simulink model "Pendulo_doble"  (R2023a)
settings: Solver=ode23  StartTime=0.0  StopTime=15  RelTol=1e-3
values from neighbouring files (symbols this model uses):
  g = 9.81    [Condiciones.mat]
  L1 = 0.3    [Condiciones.mat]
  L2 = 0.25    [Condiciones.mat]
  m1 = 0.2    [Condiciones.mat]
  m2 = 0.1    [Condiciones.mat]
settings Model: Creator=andre  LastModifiedBy=andre

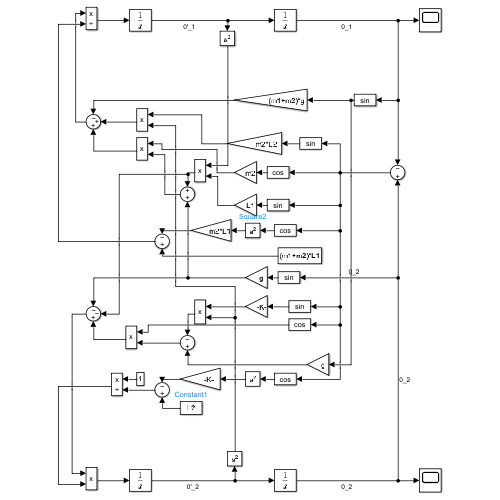
[thumbnail: Simulink's stored preview of the top-level diagram]
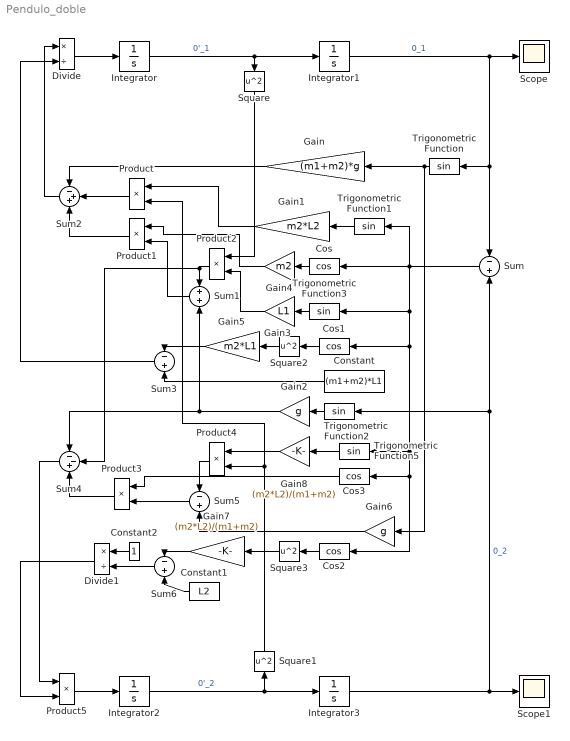
== system Pendulo_doble ==
  Constant : Constant  Value=(m1+m2)*L1
  Constant1 : Constant  Value=L2
  Constant2 : Constant
  Cos{,1..3} (4 alike) : Trigonometry  Operator=cos
  Divide : Product  Inputs=*/
  Divide1 : Product  Inputs=*/
  Gain : Gain  Gain=(m1+m2)*g
  Gain1 : Gain  Gain=m2*L2
  Gain2 : Gain  Gain=g
  Gain3 : Gain  Gain=L1
  Gain4 : Gain  Gain=m2
  Gain5 : Gain  Gain=m2*L1
  Gain6 : Gain  Gain=g
  Gain7 : Gain  Gain=(m2*L2)/(m1+m2)
  Gain8 : Gain  Gain=(m2*L2)/(m1+m2)
  Integrator : Integrator
  Integrator1 : Integrator
  Integrator2 : Integrator
  Integrator3 : Integrator  InitialCondition=35
  Product{,1..5} (6 alike) : Product
  Scope : Scope
  Scope1 : Scope
  Square{,1..3} (4 alike) : Math  Operator=square
  Sum{,3,5..6} (4 alike) : Sum  Inputs=-+
  Sum1 : Sum
  Sum2 : Sum  Inputs=-++
  Sum4 : Sum  Inputs=--+
  Trigonometric Function{,1..3,5} (5 alike) : Trigonometry
  wires:
  Integrator3/1 -> Sum/2, Trigonometric Function2/1, Scope1/1  "0_2"
  Integrator1/1 -> Sum/1, Trigonometric Function/1, Scope/1  "0_1"
  Integrator/1 -> Integrator1/1, Square/1  "0'_1"
  Integrator2/1 -> Integrator3/1, Square1/1  "0'_2"
  Sum/1 -> Cos/1, Trigonometric Function1/1, Trigonometric Function3/1, Cos2/1, Cos3/1, Trigonometric Function5/1, Cos1/1
  Trigonometric Function1/1 -> Gain1/1
  Gain1/1 -> Product/1
  Square1/1 -> Product/2, Product4/2
  Trigonometric Function2/1 -> Gain2/1
  Trigonometric Function3/1 -> Gain3/1
  Gain3/1 -> Product2/2
  Square/1 -> Product2/1
  Gain2/1 -> Sum4/1, Sum1/2
  Cos/1 -> Gain4/1
  Gain4/1 -> Product1/1
  Sum1/1 -> Product1/2
  Gain/1 -> Sum2/1
  Product/1 -> Sum2/2
  Product1/1 -> Sum2/3
  Cos1/1 -> Square2/1
  Square2/1 -> Gain5/1
  Constant/1 -> Sum3/2
  Gain5/1 -> Sum3/1
  Sum3/1 -> Divide/2
  Sum2/1 -> Divide/1
  Divide/1 -> Integrator/1
  Product2/1 -> Sum4/2, Sum1/1
  Product3/1 -> Sum4/3
  Sum5/1 -> Product3/2
  Trigonometric Function/1 -> Gain/1, Gain6/1
  Gain6/1 -> Sum5/2
  Product4/1 -> Sum5/1
  Square3/1 -> Gain7/1
  Gain7/1 -> Sum6/1
  Cos2/1 -> Square3/1
  Constant1/1 -> Sum6/2
  Product5/1 -> Integrator2/1
  Trigonometric Function5/1 -> Gain8/1
  Gain8/1 -> Product4/1
  Cos3/1 -> Product3/1
  Sum4/1 -> Product5/1
  Sum6/1 -> Divide1/2
  Constant2/1 -> Divide1/1
  Divide1/1 -> Product5/2
